simulink model "test"  (R2023a)
settings: Solver=VariableStepAuto  StartTime=0.0  StopTime=0.1  RelTol=1e-3
values from neighbouring files (symbols this model uses):
  means = [0, 0, 0]    [init.m]
  theta = [0, 0, 0]    [init.m]
  var = [1, 1, 1]    [init.m]
settings Model: Creator=lespi  LastModifiedBy=lespi
settings SolverCC: AlgebraicLoopSolver=TrustRegion
settings DataIOCC: LimitDataPoints=on  SaveOutput=off  SaveTime=off
settings OptimizationCC: BlockReduction=off  BooleanDataType=off  LifeSpan=inf
settings DebuggingCC: SaveWithParameterizedLinksMsg=none  UnderspecifiedInitializationDetection=Classic  MergeDetectMultiDrivingBlocksExec=none  SignalResolutionControl=TryResolveAllWithWarning  UnconnectedInputMsg=warning  UnconnectedOutputMsg=warning  UnconnectedLineMsg=warning  AllowSymbolicDim=off  SFUnexpectedBacktrackingDiag=warning  SFNoUnconditionalDefaultTransitionDiag=warning  SFExecutionAtInitializationDiag=none  ArithmeticOperatorsInVariantConditions=warning
settings HardwareCC: TargetUnknown=on
settings ModelReferenceCC: EnableRefExpFcnMdlSchedulingChecks=on
settings SFSimCC: SimUseLocalCustomCode=off  CustomCodeUndefinedFunction=UseInterfaceOnly
settings RTWCC: RTWUseLocalCustomCode=off
settings CodeAppCC: StateflowObjectComments=on
settings GRTTargetCC: TargetLangStandard=C89/C90 (ANSI)

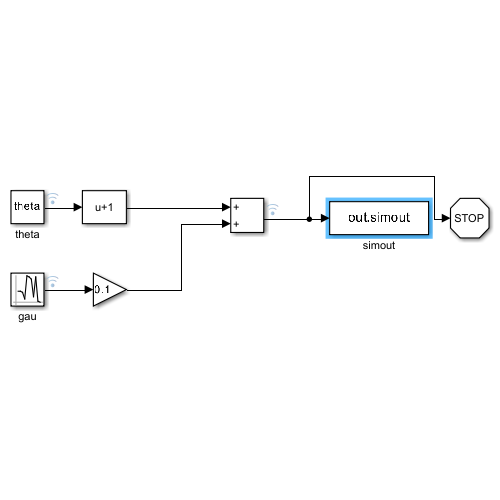
[thumbnail: Simulink's stored preview of the top-level diagram]
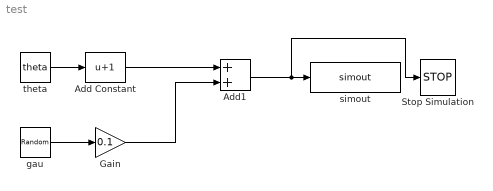
== system test ==
  Add Constant : Bias  Bias=1  SaturateOnIntegerOverflow=off
  Add1 : Sum
  Gain : Gain  Gain=0.1
  Stop Simulation : Stop
  gau : RandomNumber  Mean=means  Variance=var  Seed=10  SampleTime=0.1
  simout : ToWorkspace  VariableName=simout  SampleTime=-1
  theta : Constant  Value=theta
  wires:
  Add Constant/1 -> Add1/1
  theta/1 -> Add Constant/1
  Add1/1 -> Stop Simulation/1, simout/1
  gau/1 -> Gain/1
  Gain/1 -> Add1/2
